simulink model "ss_estimation_exact_simulink"  (R2022b)
settings: Solver=VariableStepAuto  StartTime=0.0  StopTime=10.0  RelTol=1e-3
libraries: MainLibrary x1
settings Model: Creator=cotti  LastModifiedBy=cotti

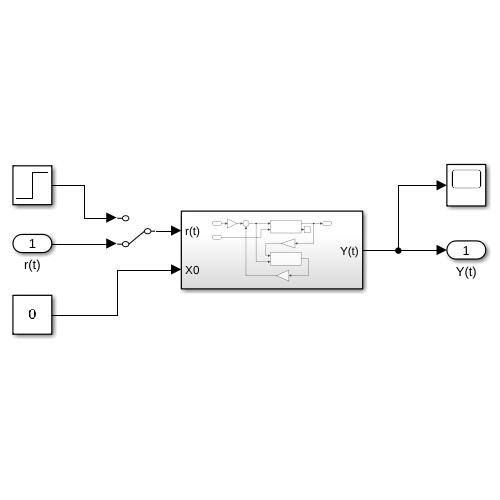
[thumbnail: Simulink's stored preview of the top-level diagram]
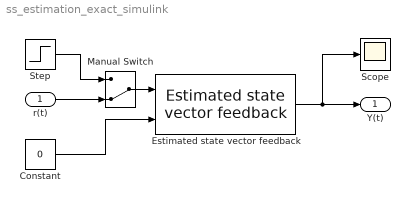
== system ss_estimation_exact_simulink ==
  r(t) : Inport
  Constant : Constant  Value=0
  Estimated state vector feedback : MainLibrary/Estimated state vector feedback  SystemSampleTime=-1  VariantActivationTime=update diagram  Latency=0  AutoFrameSizeCalculation=off
      settings: SourceProductName=Control Cotti
  Manual Switch : ManualSwitch  CurrentSetting=0
  Scope : Scope
  Step : Step  Time=0  SampleTime=0
  Y(t) : Outport
  wires:
  Estimated state vector feedback/1 -> Scope/1, Y(t)/1
  r(t)/1 -> Manual Switch/2
  Step/1 -> Manual Switch/1
  Constant/1 -> Estimated state vector feedback/2
  Manual Switch/1 -> Estimated state vector feedback/1
